simulink model "BattU_VD"  (R2016b)
settings: configuration reference "CodeGenConfigSet" (kept outside this file)
values from neighbouring files (symbols this model uses):
  BattU_facPT1_C = Calibration.Parameter    [init_BattU_VD.m]
  BattU_RmpSlpNeg_C = Calibration.Parameter    [init_BattU_VD.m]
  BattU_RmpSlpPos_C = Calibration.Parameter    [init_BattU_VD.m]
  BattU_swtRated_C = Calibration.Parameter    [init_BattU_VD.m]
  BattU_uNrm_C = Calibration.Parameter    [init_BattU_VD.m]
  BattU_uTransStgDfl_C = Calibration.Parameter    [init_BattU_VD.m]
  U_RATED_PASS = fi(14000,Battery_mv)    [init_BattU_VD.m]
  U_RATED_TRUCK = fi(28000,Battery_mv)    [init_BattU_VD.m]
undefined symbols (not defined in the file or in its folder): BattU_VD_DT, Switch_conv
libraries: CXLib x4
settings Model: Creator=Administrator  LastModifiedBy=xuxingpei
settings ConfigSetRef: SourceLocation=Base Workspace

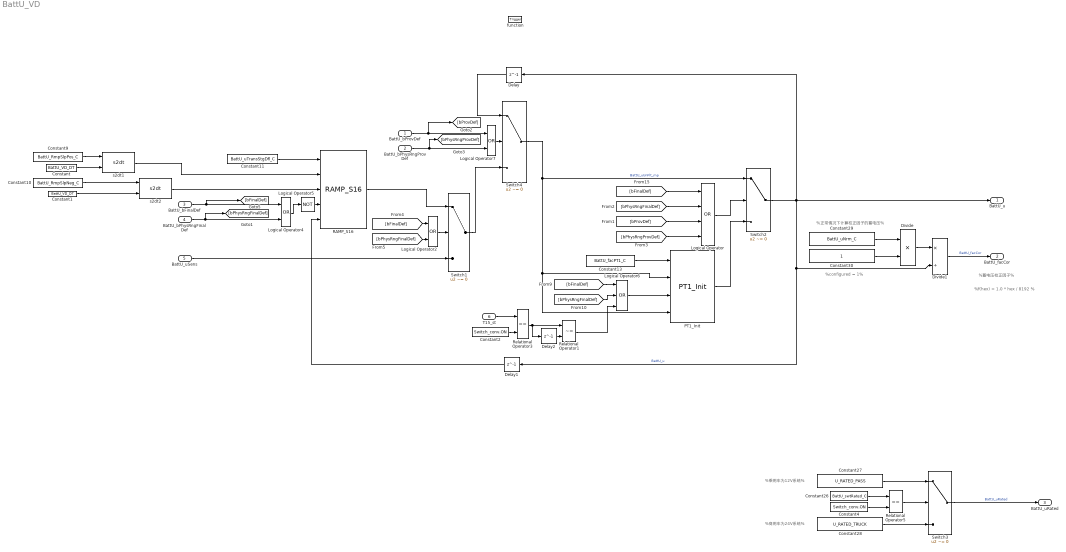
== system BattU_VD ==
  note: %configured = 1%
  note: %f(hex) = 1.0 * hex / 8192 %
  note: %正常情况下计算校正因子的蓄电压%
  note: %蓄电压校正因子%
  note: %商用车为24V系统%
  note: %乘用车为12V系统%
  BattU_bProvDef : Inport  Description=Status Sensor of the battery voltage temporary defect  OutMin=0  OutMax=1  OutDataTypeStr=boolean
  BattU_bPhysRngProvDef : Inport  Description=Status Sensor of the battery voltage physical Signal range check temporary defect  Port=2  OutMin=0  OutMax=1  OutDataTypeStr=boolean
  BattU_bFinalDef : Inport  Description=Status Sensor of the battery voltage finally defect  Port=3  OutMin=0  OutMax=1  OutDataTypeStr=boolean
  BattU_bPhysRngFinalDef : Inport  Description="Status Sensor of the  battery voltage physical Signal range check finally defect"  Port=4  OutMin=0  OutMax=1  OutDataTypeStr=boolean
  BattU_uSens : Inport  Tag=mv  Description=Sensed battery voltage  Port=5  OutMin=0  OutMax=50000  OutDataTypeStr=Battery_mv
  T15_st : Inport  Description=Terminal 15 status after debouncing  Port=6  OutDataTypeStr=Enum: Switch_conv
  function : TriggerPort  TriggerType=function-call  VariantControl=Variant
  Constant : Constant  Value=BattU_VD_DT  OutDataTypeStr=Inherit: Inherit via back propagation
  Constant1 : Constant  Value=BattU_VD_DT  OutDataTypeStr=Inherit: Inherit via back propagation
  Constant10 : Constant  Value=BattU_RmpSlpNeg_C  SampleTime=-1
  Constant11 : Constant  Value=BattU_uTransStgDfl_C  SampleTime=-1
  Constant13 : Constant  Value=BattU_facPT1_C  SampleTime=-1
  Constant2 : Constant  Value=Switch_conv.ON
  Constant26 : Constant  Value=BattU_swtRated_C  SampleTime=-1
  Constant27 : Constant  Value=U_RATED_PASS  SampleTime=-1
  Constant28 : Constant  Value=U_RATED_TRUCK  SampleTime=-1
  Constant29 : Constant  Value=BattU_uNrm_C  SampleTime=-1
  Constant30 : Constant  OutDataTypeStr=Factor  SampleTime=-1
  Constant4 : Constant  Value=Switch_conv.ON  OutDataTypeStr=Inherit: Inherit via back propagation
  Constant9 : Constant  Value=BattU_RmpSlpPos_C  SampleTime=-1
  Delay : Delay  DialogController=Simulink.DDGSource  DelayLength=1  InitialCondition=0
  Delay1 : Delay  DialogController=Simulink.DDGSource  DelayLength=1  InitialCondition=0
  Delay2 : Delay  DelayLength=1  InitialCondition=0
  Divide : Product  Inputs=**  OutDataTypeStr=Battery_mv  SaturateOnIntegerOverflow=on
  Divide1 : Product  Inputs=*/  OutDataTypeStr=Factor  SaturateOnIntegerOverflow=on
  Logical Operator : Logic  Operator=OR  Inputs=4  OutDataTypeStr=boolean
  Logical Operator2 : Logic  Operator=OR  OutDataTypeStr=boolean
  Logical Operator4 : Logic  Operator=OR  OutDataTypeStr=boolean
  Logical Operator5 : Logic  Operator=NOT  AllPortsSameDT=off  OutDataTypeStr=boolean
  Logical Operator6 : Logic  Operator=OR  Inputs=3  OutDataTypeStr=boolean
  Logical Operator7 : Logic  Operator=OR  OutDataTypeStr=boolean
  PT1_Init : CXLib/PT1_Init
  RAMP_S16 : CXLib/RAMP_S16
  Relational Operator1 : RelationalOperator  Operator=~=  OutDataTypeStr=boolean  RndMeth=Simplest
  Relational Operator3 : RelationalOperator  Operator===  OutDataTypeStr=boolean  RndMeth=Simplest
  Relational Operator5 : RelationalOperator  Operator===  OutDataTypeStr=boolean  RndMeth=Simplest  InputSameDT=on
  Switch1 : Switch  Criteria=u2 ~= 0  InputSameDT=on
  Switch2 : Switch  Criteria=u2 ~= 0  InputSameDT=on
  Switch3 : Switch  Criteria=u2 ~= 0  OutDataTypeStr=Inherit: Inherit via back propagation  InputSameDT=on
  Switch4 : Switch  Criteria=u2 ~= 0  InputSameDT=on
  s2dt1 : CXLib/s2dt
  s2dt2 : CXLib/s2dt
  BattU_u : Outport  Tag=mv  Description=Battery voltage  OutMin=0  OutMax=50000  OutDataTypeStr=Battery_mv
  BattU_facCor : Outport  Description=Battery correction factor  Port=2  OutMin=-32  OutMax=31.9  OutDataTypeStr=Factor
  BattU_uRated : Outport  Tag=mv  Description=Rated battery voltage  Port=3  OutMin=0  OutMax=50000  OutDataTypeStr=Battery_mv
  wires:
  BattU_uSens/1 -> Switch1/3
  Delay/1 -> Switch4/1
  Switch4/1 -> PT1_Init/2, PT1_Init/4, Switch2/1  "BattU_uUnFlt_mp"
  Switch1/1 -> Switch4/3
  Logical Operator/1 -> Switch2/2
  Switch2/1 -> BattU_u/1, Delay/1, Delay1/1, Divide1/2  "BattU_u"
  Logical Operator7/1 -> Switch4/2
  Logical Operator2/1 -> Switch1/2
  Logical Operator4/1 -> Logical Operator5/1
  s2dt1/1 -> RAMP_S16/2
  s2dt2/1 -> RAMP_S16/3
  Constant13/1 -> PT1_Init/1
  Constant11/1 -> RAMP_S16/1
  RAMP_S16/1 -> Switch1/1
  PT1_Init/1 -> Switch2/3
  BattU_bProvDef/1 -> [bProvDef], Logical Operator7/1
  BattU_bPhysRngProvDef/1 -> [bPhysRngProvDef], Logical Operator7/2
  [bFinalDef] -> Logical Operator/1
  [bPhysRngFinalDef] -> Logical Operator/2
  [bProvDef] -> Logical Operator/3
  [bPhysRngProvDef] -> Logical Operator/4
  [bFinalDef] -> Logical Operator2/1
  [bPhysRngFinalDef] -> Logical Operator2/2
  Logical Operator5/1 -> RAMP_S16/4
  [bFinalDef] -> Logical Operator6/1
  [bPhysRngFinalDef] -> Logical Operator6/2
  Logical Operator6/1 -> PT1_Init/3
  BattU_bPhysRngFinalDef/1 -> Logical Operator4/2, [bPhysRngFinalDef]
  BattU_bFinalDef/1 -> Logical Operator4/1, [bFinalDef]
  Constant29/1 -> Divide/1
  Constant30/1 -> Divide/2
  Divide/1 -> Divide1/1
  Divide1/1 -> BattU_facCor/1  "BattU_facCor"
  Relational Operator5/1 -> Switch3/2
  Constant26/1 -> Relational Operator5/1
  Constant27/1 -> Switch3/1
  Constant28/1 -> Switch3/3
  Switch3/1 -> BattU_uRated/1  "BattU_uRated"
  Constant4/1 -> Relational Operator5/2
  Constant9/1 -> s2dt1/1
  Constant/1 -> s2dt1/2
  Constant10/1 -> s2dt2/1
  Constant1/1 -> s2dt2/2
  Delay1/1 -> RAMP_S16/5
  Constant2/1 -> Relational Operator3/2
  Delay2/1 -> Relational Operator1/2
  Relational Operator3/1 -> Delay2/1, Relational Operator1/1
  Relational Operator1/1 -> Logical Operator6/3
  T15_st/1 -> Relational Operator3/1
